simulink model "spring_damping_mass_System_1dof"  (R2013b)
settings: Solver=ode45  StartTime=0.0  StopTime=10.0  RelTol=1e-3
undefined symbols (not defined in the file): c, k, m
settings Model: Creator=edward  LastModifiedBy=edward

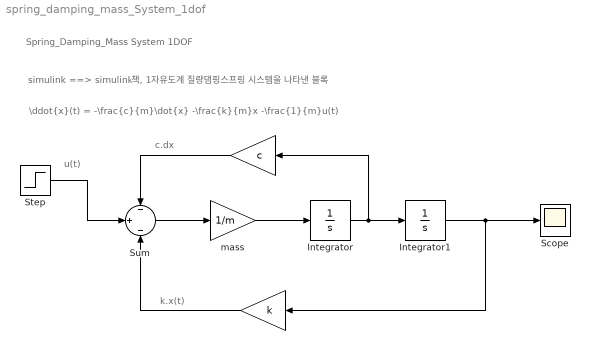
== system spring_damping_mass_System_1dof ==
  note: \ddot{x}(t) = -\frac{c}{m}\dot{x} -\frac{k}{m}x -\frac{1}{m}u(t)
  note: simulink ==> simulink책, 1자유도계 질량댐핑스프링 시스템을 나타낸 블록
  note: Spring_Damping_Mass System 1DOF
  note: u(t)
  note: k.x(t)
  note: c.dx
  " " : Gain  Gain=c
  " " : Gain  Gain=k
  Integrator : Integrator
  Integrator1 : Integrator
  Scope : Scope
  Step : Step  Time=0  SampleTime=0
  Sum : Sum  Inputs=-|+|-
  "mass " : Gain  Gain=1/m
  wires:
  Integrator1/1 -> Scope/1, " "/1
  Sum/1 -> "mass "/1
  Integrator/1 -> Integrator1/1, " "/1
  "mass "/1 -> Integrator/1
  " "/1 -> Sum/3
  " "/1 -> Sum/1
  Step/1 -> Sum/2
